simulink model "SpeedgoatCANOpen2Buses1ms"  (R2018b)
settings: Solver=ode8  StartTime=0.0  StopTime=inf  FixedStep=0.001  RelTol=1e-3  EnableMultiTasking=on
undefined symbols (not defined in the file or in its folder): DiscIntNeverNeededParam
libraries: slrtlib x6, speedgoatlib_IO691 x5, dspstat3 x5, simulink x5
(part 3 of 3)

== stateflow chart SpeedgoatCANOpen2Buses1ms/Trike Application Layer/System_Init/EnableCtrl ==
  state Init
    du:
    Enable    =  1;
  state Enable_Control
    du:
    Enable    =  1;
  (default) -> Init
  Init -> Enable_Control : [ButtonStatus == 6 ]
  Enable_Control -> Init : [ButtonStatus == 7 ]
  data: ButtonStatus input single; Enable output single

== stateflow chart SpeedgoatCANOpen2Buses1ms/Trike Application Layer/System_Control/BrakeControl/Subsystem/Retract ==
  state Init
    entry:
    Br_CurrentReq = 0;
  state Retract
    du:
    Br_CurrentReq = 1;
  (default) -> Init
  Init -> Retract : [PedalTravelGradient > 0.05 ]
  Retract -> Init : [after(500,tick)]
  data: PedalTravelGradient input single; Br_CurrentReq output single; PedalTravel input single

== matlab function SpeedgoatCANOpen2Buses1ms/Trike Application Layer/System_Control/BrakeControl/MATLAB Function ==
  data: LongCmd input; ButtonStatus input; button output
function button = JoystickButtonStatus(LongCmd, ButtonStatus)
aux = 0;
aux2 = 0;

if LongCmd <= 0
    aux2 = - double (LongCmd);
else 
    aux2 = 0;
end
switch (ButtonStatus)
    case 4
        aux = 1;
    case 8
        aux = 1;
    case 16
        aux = 1;
        aux2 = 500;
    otherwise
        aux = 0;
end
button =aux * aux2;

== matlab function SpeedgoatCANOpen2Buses1ms/Inclinometer_RPDOs/Conv ==
  data: xSign input uint8; xAngle output double; xAngleH input uint8; xAngleL input uint8; ySign input uint8; yAngleH input uint8; yAngleL input uint8; yAngle output double
function [xAngle,yAngle] = Angle(xSign,xAngleH,xAngleL,ySign,yAngleH,yAngleL)
if xSign == 0
    aux_xSign=1;
else    
    aux_xSign=-1;
end
if ySign == 0
    aux_ySign=1;
else    
    aux_ySign=-1;
end

xAngle = aux_xSign * real(str2double(dec2hex(xAngleH))+str2double(dec2hex(xAngleL))/100);
yAngle = aux_ySign * real(str2double(dec2hex(yAngleH))+str2double(dec2hex(yAngleL))/100);

== matlab function SpeedgoatCANOpen2Buses1ms/Trike Application Layer/System_Control/TiltingControl/PID_ctrl1/Derivative ==
  data: y input; ud output; yf output
function [ud,yf]  = deriv(y)

Ts = 0.015;
Tf = 0.20; 
Kd = 0.2; 
  c0    = Ts / (Ts + Tf);
persistent yf_k1

if isempty(yf_k1)     
    yf_k1 = single(0);    
end

yf = yf_k1 + c0 * (y - yf_k1);
ud = Kd * (yf - yf_k1) / Ts ; 

yf_k1 = yf;

== matlab function SpeedgoatCANOpen2Buses1ms/Trike Application Layer/System_Control/SteeringControl/P Controller ==
  data: DirectionReq input; SpeedReq output; DirectionFb input
function SpeedReq  = fcn(DirectionReq,DirectionFb)


if (DirectionReq>90)
    DirectionReq=90;
end
if (DirectionReq<-90)
    DirectionReq=-90;
end
err = DirectionReq - DirectionFb;

Kp = 70;

SpeedReq = Kp * err;  


end

== matlab function SpeedgoatCANOpen2Buses1ms/Trike Application Layer/System_Control/TiltingControl/TiltingController/PID_Incremental_V1/PI_incremental Tilting Controller ==
  data: PosRef input; LTiltCurrRef output; Pos input; RTiltCurrRef output; En input; up output; ui output; ud output
function [LTiltCurrRef, RTiltCurrRef,up,ui,ud] = fcn(PosRef,Pos,En)
persistent uk1 ek1 udk1 Posk1
if (isempty(uk1))
    Posk1 = 0;
    udk1 = 0;
    uk1 = 0;
    ek1 = 0; 
end

% +/- 0.076 m
pos_lim = 0.02;
imax = 10;


if En == 0
    
    u = 0;
    Kp = 0;
    Ki = 0;
    Kd = 0;
else
    
    Kp = 1200;  % 800 pt 1ms
    Ki = 3;     % 5
    Kd = 2;     % 5
    
end


if (PosRef > pos_lim)
    PosRef = pos_lim;
end
if (PosRef <- pos_lim)
   PosRef = -pos_lim;
end

e = PosRef - Pos;

Te = 0.005;
up = Kp * (e - ek1);
ui = Ki * e;
ud = -udk1 - Kd * (Pos - Posk1)*2/Te;


Du = up + ui + ud;

u = uk1 + Du;

if (u > imax)
    u = imax;
end
if (u<-imax)
    u=-imax;
end

LTiltCurrRef =  u;
RTiltCurrRef = -u;

Posk1 = Pos;
udk1  = ud;
uk1   = u;
ek1   = e;

== matlab function SpeedgoatCANOpen2Buses1ms/Trike Application Layer/System_Control/TiltingControl/ServoTilting ==
  data: SteerAngle input; VehSpeed_SI input; TiltingAngle output
function TiltingAngle  = CalcTiltAngle(SteerAngle,VehSpeed_SI)
%SteerAngle [rad]
%TravelingSpeed [m/s]
L = 1.025;
g = 9.81;
TiltingAngle = atan(VehSpeed_SI^2/(L*g)*sin(SteerAngle));
TiltingAngle = TiltingAngle *180/pi;
% TiltingAngle [deg]

== stateflow chart SpeedgoatCANOpen2Buses1ms/Trike Application Layer/System_Init/Steering_DunkMotor_Init/DunkA_Steering_Init_SpeedMode ==
  state Init
    entry:
    ClearError       = 0;
    DeviceMode   = 0;
    BrakeCtrl        = 0;
    PowerEnable = 0;
    aux                 = 0;
    InitStatus        = 0;
  state Clear_Error
    du:
    ClearError = 1;
    aux            = aux + 1;
    InitStatus   = 0;
  state Wait
    en:
    BrakeCtrl = 2;
    aux          = aux + 1;
    InitStatus = 0;
  state SetCurrentMode
    du:
    DeviceMode  = 3; % SpeedMode
    PowerEnable = 1;
    InitStatus       = 1;
  (default) -> Init
  Init -> Clear_Error : %[ButtonStatus == 1 ||...
      | % ReadError ~= 1]
  Clear_Error -> Wait : [aux > 40000]{aux = 0;}
  (junction 262) -> Init
  Wait -> Wait [order 1] : [aux < 20 && ReadError == 1]
  Wait -> (junction 262) [order 3] : [ReadError ~= 1]
  (junction 264) -> (junction 262)
  Wait -> SetCurrentMode [order 2] : [aux >= 20 && ReadError == 1]{aux = 0;}
  SetCurrentMode -> (junction 264) : [ReadError ~= 1]
  data: ButtonStatus input single; ClearError output single; DeviceMode output single; BrakeCtrl output single; ReadError input single; aux2 local single; aux local single; PowerEnable output single; InitStatus output single

== stateflow chart SpeedgoatCANOpen2Buses1ms/Trike Application Layer/System_Control/BrakeControl/DecisionBrakeCtrl ==
  state Init
    entry:
    BrakesMotor_CurrentReq = 0;
    BrakeCtrl          = BrakeCtrlIn;
    Parking_Brake =  0;
    Neutral_State   =  0;
  state %Parking_Break
    entry:
    BrakeCtrl     = 2;
    BrakesMotor_CurrentReq = -10000;
    Parking_Brake =1;
    Neutral_State =0;
  state %Neutral state [commented out]
    entry:
    BrakeCtrl     = 0;
    BrakesMotor_CurrentReq = 0;
    Neutral_State = 1;
    Parking_Brake = 0;
  (default) -> Init
  %Parking_Break -> Init : [BrakesMotor_CurrentReqIn < 10 &&...
      | BrakesMotor_CurrentReqIn > -10]
  (junction 284) -> %Parking_Break [commented out] : [Neutral_State == 1 &&  JsButton == 3]
  Init -> %Parking_Break : [BrakesMotor_CurrentReqIn > 100 ||...
      | BrakesMotor_CurrentReqIn < -100]
  %Parking_Break -> (junction 273) [commented out] : after(500, msec)
  (junction 273) -> %Neutral state [commented out] : [Parking_Brake == 1 && JsButton == 4 ]
  %Neutral state -> (junction 284) [commented out] : after(500, msec)
  data: BrakesMotor_CurrentReqIn input; VehSpeed input; BrakesMotor_CurrentReq output; BrakeCtrlIn input; BrakeCtrl output; JsButton input; JsLongCmd input; Neutral_State local; Parking_Brake local

== matlab function SpeedgoatCANOpen2Buses1ms/Trike Application Layer/System_Init/ButtonStatus ==
  data: ButtonStatus input; Button output
function Button = JoystickButtonStatus(ButtonStatus)
aux = 0;
switch (ButtonStatus)
    case 1
        aux = 1;
    case 2
        aux = 2;
    case 4
        aux = 3;
    case 8
        aux = 4;
    case 16
        aux = 5;
    case 32
        aux = 6; 
    case 64
        aux = 7;
    case 128 
        aux = 8;
    otherwise
        aux = 0;
end
Button =aux;

== matlab function SpeedgoatCANOpen2Buses1ms/Trike Application Layer/CAN_B/HeartBeatgenerator ==
  data: HB output
function HB = HBGenerator
persistent tact Heartbeat
if (isempty(Heartbeat))
    Heartbeat = 0;
    tact = 0;
end
tact=tact+1;
if (tact>10)
    tact=0;
    Heartbeat=Heartbeat+1;
    if (Heartbeat>127)
        Heartbeat = 0;    
    end
end
HB = Heartbeat;

== matlab function SpeedgoatCANOpen2Buses1ms/Trike Application Layer/System_Init/APTControlWord ==
  data: ButtonStatus input; APT_CtrlWord output; LongCmd input
function APT_CtrlWord = TractionCtrl(ButtonStatus, LongCmd)
Direction =0;
if (ButtonStatus==8)
    if(LongCmd>0)
        Direction = 4;
    elseif (LongCmd<0)
        Direction = 8;
    end
 end
APT_CtrlWord =160+Direction;
